simulink model "rtwdemo_capi"  (Simulink 6.0)
settings: Solver=FixedStepDiscrete  StartTime=0.0  StopTime=10.0  RelTol=1e-3
PostLoadFcn:
  | rtwdemo_capi_data
values from neighbouring files (symbols this model uses):
  Ki = Simulink.Parameter    [rtwdemo_capi_data.m]
  Kp = Simulink.Parameter    [rtwdemo_capi_data.m]
  p1 = Simulink.Parameter    [rtwdemo_capi_data.m]
  p2 = Simulink.Parameter    [rtwdemo_capi_data.m]
  p3 = Simulink.Parameter    [rtwdemo_capi_data.m]
libraries: rtwdemowidgets x4, simulink x3
settings Model: Creator=The MathWorks Inc.  LastModifiedBy=batserve  ExtModeTrigMode=oneshot  ExtModeArmWhenConnect=off  ExtModeAutoUpdateStatusClock=off
settings DataIOCC: LimitDataPoints=off  SaveFormat=Structure  SaveOutput=off  SaveTime=off  SignalLoggingName=sigsOut
settings OptimizationCC: InlineParams=on  EnforceIntegerDowncast=off  StateBitsets=on  DataBitsets=on  UseTempVars=on
settings DebuggingCC: CheckExecutionContextPreStartOutputMsg=on  CheckExecutionContextRuntimeOutputMsg=on  SignalResolutionControl=TryResolveAll  SolverPrmCheckMsg=none  UnconnectedInputMsg=none  UnconnectedOutputMsg=none  UnconnectedLineMsg=none
settings RTWCC: TLCOptions=-p0 -aWarnNonSaturatedBlocks=0  GenCodeOnly=on  GenerateReport=on  RTWVerbose=off  ProcessScript=grt_make_rtw_hook  LaunchReport=on
settings CodeAppCC: ForceParamTrailComments=on  PrefixModelToSubsysFcnNames=off
settings GRTTargetCC: RTWCAPISignals=on  RTWCAPIParams=on

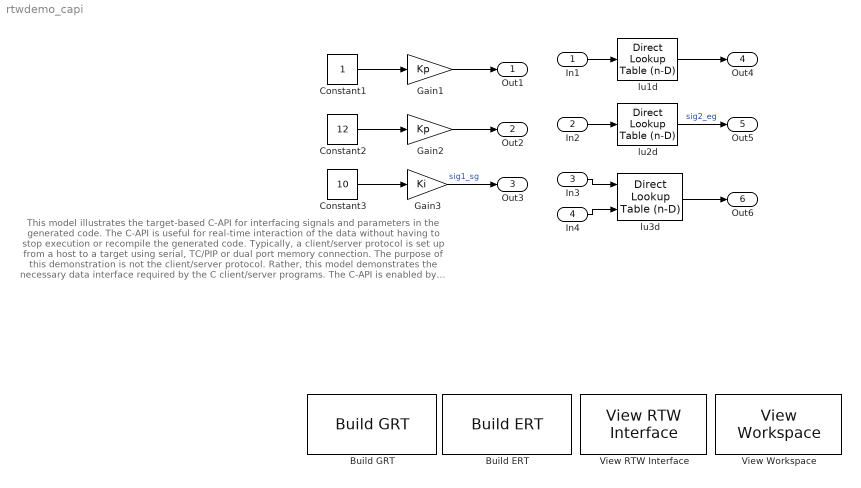
== system rtwdemo_capi ==
  note: This model illustrates the target-based C-API for interfacing signals and parameters in the generated code.  The
      | C-API is useful for real-time interaction of the data without having to stop execution or recompile the
      | generated code.  Typically, a client/server protocol is set up from a host to a target using serial, TC/PIP or
      | dual port memory connection.  The purpose of this demonstration is not the client/server protocol.  Rather, this
      | model demonstrates the necessary data interface required by the C client/server programs.
      |
      | The C-API is enabled by the Real-Time Workshop option "Data Exchange" set to C-API.  Any signal or parameter
      | with an addressable storage class is placed in the C-API data structure located in <model>_capi.c.
  In1 : Inport  Port=1  LatchInput=off
  In2 : Inport  Port=2  LatchInput=off
  In3 : Inport  Port=3  LatchInput=off
  In4 : Inport  Port=4  LatchInput=off
  Build ERT : rtwdemowidgets/Build ERT  attrib_overrides={'RTWCAPIParams','RTWCAPISignals'}
  Build GRT : rtwdemowidgets/Build GRT  attrib_overrides={'RTWCAPIParams','RTWCAPISignals'}
  Constant1 : Constant
  Constant2 : Constant  Value=12
  Constant3 : Constant  Value=10
  Gain1 : Gain  Gain=Kp  SaturateOnIntegerOverflow=on
  Gain2 : Gain  Gain=Kp  SaturateOnIntegerOverflow=on
  Gain3 : Gain  Gain=Ki  SaturateOnIntegerOverflow=on
  View RTW Interface : rtwdemowidgets/View RTW Interface
  View Workspace : rtwdemowidgets/View Workspace
  lu1d : simulink/Lookup Tables/Direct Lookup Table (n-D)  Priority=5  maskTabDims=1  explicitNumDims=1  outDims=Element  tabIsInput=off  mxTable=p1  clipFlag=Warning
  lu2d : simulink/Lookup Tables/Direct Lookup Table (n-D)  Priority=6  maskTabDims=2  explicitNumDims=1  outDims=Column  tabIsInput=off  mxTable=p2  clipFlag=Warning
  lu3d : simulink/Lookup Tables/Direct Lookup Table (n-D)  Priority=7  maskTabDims=3  explicitNumDims=1  outDims=Column  tabIsInput=off  mxTable=p3  clipFlag=Warning
  Out1 : Outport
  Out2 : Outport  Port=2
  Out3 : Outport  Port=3
  Out4 : Outport  Port=4
  Out5 : Outport  Port=5
  Out6 : Outport  Port=6
  wires:
  Gain1/1 -> Out1/1
  Constant1/1 -> Gain1/1
  Gain2/1 -> Out2/1
  Constant2/1 -> Gain2/1
  Gain3/1 -> Out3/1  "sig1_sg"
  Constant3/1 -> Gain3/1
  lu1d/1 -> Out4/1
  lu2d/1 -> Out5/1  "sig2_eg"
  lu3d/1 -> Out6/1
  In1/1 -> lu1d/1
  In2/1 -> lu2d/1
  In3/1 -> lu3d/1
  In4/1 -> lu3d/2
